simulink model "untitled111"  (Simulink 8.2)
settings: Solver=ode45  StartTime=0.0  StopTime=.06  RelTol=1e-3
libraries: powerlib x42
settings Model: Creator=Pratp_000  LastModifiedBy=Pratp_000
settings DataIOCC: SignalLoggingSaveFormat=Dataset
settings OptimizationCC: ExpressionDepthLimit=128
settings DebuggingCC: FcnCallInpInsideContextMsg=EnableAllAsError  StateNameClashWarn=none
settings GRTTargetCC: CombineOutputUpdateFcns=on  GRTInterface=off

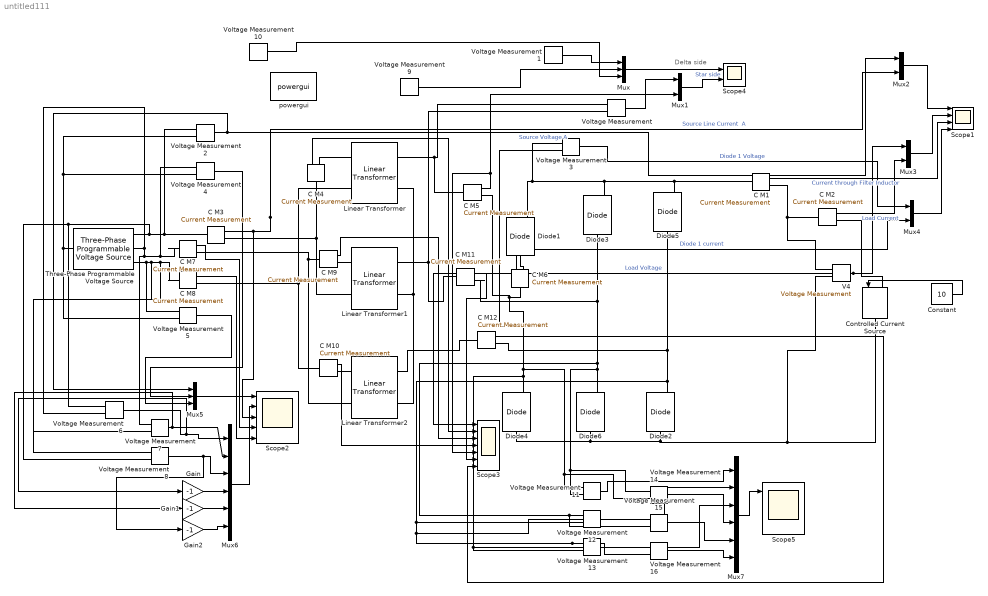
== system untitled111 ==
  note: Delta side
  C M{1..12} (12 alike) : powerlib/Measurements/Current Measurement  PhasorSimulation=off  OutputType=Complex  PSBequivalent=0
  Constant : Constant  Value=10
  Controlled Current Source : powerlib/Electrical Sources/Controlled Current Source  Initialize=on  Source_Type=DC  Amplitude=10  Phase=0  Frequency=0  Measurements=None
  Diode{1..6} (6 alike) : powerlib/Power Electronics/Diode  Ron=0.001  Lon=0  Vf=0.8  IC=0  UseSnubber=off  Rs=500  Cs=250e-9  Measurements=on
  Gain : Gain  Gain=-1
  Gain1 : Gain  Gain=-1
  Gain2 : Gain  Gain=-1
  Linear Transformer : powerlib/Elements/Linear Transformer  UNITS=pu  NominalPower=[ 84e3 50 ]  winding1="[ 440  0.00  0.0 ]"  winding2="[ 254.034  0.00  0.0 ]"  ThreeWindings=off  winding3=[ 315e3 0.002 0.08 ]  RmLm=[ 0 000 ]  Measurements=None  DataType=off
  Linear Transformer1 : powerlib/Elements/Linear Transformer  UNITS=pu  NominalPower=[ 84e3 50 ]  winding1="[ 440  0.00  0.0 ]"  winding2="[ 254.034  0.00  0.0 ]"  ThreeWindings=off  winding3=[ 315e3 0.002 0.08 ]  RmLm=[ 0 0 ]  Measurements=None  DataType=off
  Linear Transformer2 : powerlib/Elements/Linear Transformer  UNITS=pu  NominalPower=[ 84e3 50 ]  winding1="[ 440  0.00  0.0 ]"  winding2="[ 254.034  0.00  0.0 ]"  ThreeWindings=off  winding3=[ 315e3 0.002 0.08 ]  RmLm=[ 00 00 ]  Measurements=None  DataType=off
  Mux : Mux  Inputs=3
  Mux{1..4} (4 alike) : Mux  Inputs=2
  Mux5 : Mux  Inputs=3
  Mux6 : Mux  Inputs=6
  Mux7 : Mux  Inputs=6
  Scope1 : Scope  NumInputPorts=4
      settings: ShowLegends=on  YMin=0~-5~-5~-5  YMax=50~5~5~5  Decimation=3
  Scope2 : Scope  NumInputPorts=5
      settings: YMin=-200~-350~-0.459708~-2.18199~2.39011  YMax=200~200~-0.415926~-1.97419~2.64171  SaveName=pp  Decimation=3
  Scope3 : Scope  NumInputPorts=7
      settings: YMin=0~-5~-5~-5~-5~-5~-5  YMax=50~5~5~5~5~5~5  SaveName=pp2  Decimation=3
  Scope4 : Scope  NumInputPorts=2
      settings: YMin=0~-5  YMax=50~5  SaveName=pp4  Decimation=3
  Scope5 : Scope  NumInputPorts=6
      settings: YMin=-200~-350~-0.459708~-2.18199~2.39011~-5  YMax=200~200~-0.415926~-1.97419~2.64171~5  SaveName=pp1  Decimation=3
  Three-Phase Programmable Voltage Source : powerlib/Electrical Sources/Three-Phase Programmable Voltage Source  PositiveSequence="[220  0 50]"  VariationEntity=None  VariationType=Table of time-amplitude pairs  VariationTypeAlt=Step  VariationStep=0.5  VariationRate=10  VariationMagnitude=0.3  VariationFrequency=2  VariationTiming=[1 2]  VariationPhaseA=off  Amplitudes=[1 0.8 1.2 1.0]  TimeValues=[0 0.1 0.15 0.2]  HarmonicGeneration=off  HarmonicA=[3 0.2 -25 0]  HarmonicB=[2 0.15 35 2]  Timing="[0.05  3]"  BusType=swing  Pref=0  Qref=0  Qmin=-inf  Qmax=inf
  V4 : powerlib/Measurements/Voltage Measurement  PhasorSimulation=off  OutputType=Complex  PSBequivalent=0
  Voltage Measurement{,1..16} (17 alike) : powerlib/Measurements/Voltage Measurement  PhasorSimulation=off  OutputType=Complex  PSBequivalent=0
  powergui : powerlib/powergui  Priority=1  SimulationMode=Discrete  SolverType=Tustin  SampleTime=10e-6  frequency=60  SPID=off  DisableSnubberDevices=off  DisableRonSwitches=off  DisableVfSwitches=off  SwTol=0  Interpol=off  DisplayEquations=off  frequencyindice=50  Pbase=100e6  ErrMax=1e-4  Iterations=50  UnitsV=kV  UnitsW=MW  FunctionMessages=off  echomessages=off  HookPort=off  EnableUseOfTLC=off  x0status=blocks  RestoreLinks=warning  ResistiveCurrentMeasurement=off  Frange=[0:2:500]  Ylog=off  Xlog=on  ShowGrid=off  save=off  variable=ZData  structure=ScopeData1  ZoomFFT=on  StartTime=0.1  cycles=1  DisplayStyle=1  fundamental=50  FreqAxis=on  MaxFrequency=1000  frequencyindicesteady=1  RmsSteady=1  display=off  Ts=0  methode=off
  wires:
  Mux/1 -> Scope4/1
  Voltage Measurement1/1 -> Mux/1
  Voltage Measurement2/1 -> Mux5/1, Mux2/1  "Source Voltage A"
  C M3/1 -> Scope2/3, Mux2/2  "Source Line Current  A"
  C M2/1 -> Mux3/2  "Load Current"
  V4/1 -> Mux3/1, Scope3/1  "Load Voltage"
  C M4/1 -> Scope3/2
  Voltage Measurement/1 -> Mux1/1
  C M5/1 -> Scope3/5, Mux1/2
  Mux1/1 -> Scope4/2  "Star side"
  Mux2/1 -> Scope1/1
  Mux3/1 -> Scope1/2
  C M1/1 -> Scope1/3  "Current through Filter Inductor"
  Voltage Measurement3/1 -> Mux4/1  "Diode 1 Voltage"
  Mux4/1 -> Scope1/4
  C M6/1 -> Mux4/2  "Diode 1 current"
  Voltage Measurement4/1 -> Mux5/2
  Voltage Measurement5/1 -> Mux5/3
  Mux5/1 -> Scope2/1
  Voltage Measurement6/1 -> Gain/1, Mux6/1
  Voltage Measurement7/1 -> Gain1/1, Mux6/2
  Voltage Measurement8/1 -> Gain2/1, Mux6/3
  Mux6/1 -> Scope2/2
  C M7/1 -> Scope2/4
  C M8/1 -> Scope2/5
  Constant/1 -> Controlled Current Source/1
  C M9/1 -> Scope3/3
  C M10/1 -> Scope3/4
  C M12/1 -> Scope3/7
  C M11/1 -> Scope3/6
  Voltage Measurement9/1 -> Mux/2
  Voltage Measurement10/1 -> Mux/3
  Gain2/1 -> Mux6/6
  Gain1/1 -> Mux6/5
  Gain/1 -> Mux6/4
  Voltage Measurement11/1 -> Mux7/1
  Voltage Measurement12/1 -> Mux7/2
  Voltage Measurement13/1 -> Mux7/3
  Voltage Measurement14/1 -> Mux7/4
  Voltage Measurement15/1 -> Mux7/5
  Voltage Measurement16/1 -> Mux7/6
  Mux7/1 -> Scope5/1
  connections:
  Linear Transformer2/RConn2 -- Linear Transformer/RConn2 -- Linear Transformer1/RConn2
  Voltage Measurement/LConn1 -- C M5/LConn1 -- Linear Transformer/RConn1
  C M11/RConn1 -- Diode3/LConn1 -- Voltage Measurement15/LConn2 -- Voltage Measurement12/LConn1 -- Voltage Measurement14/LConn1 -- Voltage Measurement11/LConn2 -- Diode6/RConn1
  C M12/RConn1 -- Diode5/LConn1 -- Voltage Measurement16/LConn2 -- Voltage Measurement13/LConn1 -- Voltage Measurement15/LConn1 -- Voltage Measurement12/LConn2 -- Diode2/RConn1
  Diode4/LConn1 -- Diode6/LConn1 -- Controlled Current Source/RConn1 -- V4/LConn2 -- Diode2/LConn1
  C M1/RConn1 -- V4/LConn1 -- C M2/LConn1
  C M2/RConn1 -- Controlled Current Source/LConn1
  Voltage Measurement2/LConn2 -- Voltage Measurement5/LConn2 -- Three-Phase Programmable Voltage Source/LConn1 -- Voltage Measurement4/LConn2
  Voltage Measurement2/LConn1 -- C M3/LConn1 -- Voltage Measurement8/LConn2 -- Voltage Measurement6/LConn1 -- Three-Phase Programmable Voltage Source/RConn1
  Diode1/LConn1 -- C M6/RConn1
  C M6/LConn1 -- Voltage Measurement3/LConn2 -- Voltage Measurement14/LConn2 -- Voltage Measurement11/LConn1 -- Voltage Measurement16/LConn1 -- Voltage Measurement13/LConn2 -- Diode4/RConn1 -- C M5/RConn1
  C M7/LConn1 -- Voltage Measurement4/LConn1 -- Voltage Measurement7/LConn1 -- Voltage Measurement6/LConn2 -- Three-Phase Programmable Voltage Source/RConn2
  C M8/LConn1 -- Voltage Measurement8/LConn1 -- Voltage Measurement7/LConn2 -- Voltage Measurement5/LConn1 -- Three-Phase Programmable Voltage Source/RConn3
  C M11/LConn1 -- Linear Transformer1/RConn1 -- Voltage Measurement/LConn2
  Linear Transformer2/RConn1 -- C M12/LConn1
  Diode1/RConn1 -- Voltage Measurement3/LConn1 -- Diode3/RConn1 -- C M1/LConn1 -- Diode5/RConn1
  Linear Transformer/LConn1 -- C M4/RConn1
  C M4/LConn1 -- C M3/RConn1 -- Linear Transformer1/LConn2
  Linear Transformer1/LConn1 -- C M9/RConn1
  C M9/LConn1 -- Linear Transformer2/LConn2 -- C M7/RConn1
  Linear Transformer2/LConn1 -- C M10/RConn1
  C M10/LConn1 -- C M8/RConn1 -- Linear Transformer/LConn2
